simulink model "Tie_Line_bias"  (R2020a)
settings: Solver=VariableStepAuto  StartTime=0.0  StopTime=30  MaxStep=1e-4  RelTol=1e-3
libraries: powerlib x1
settings Model: Creator=Zebin  LastModifiedBy=Zebin

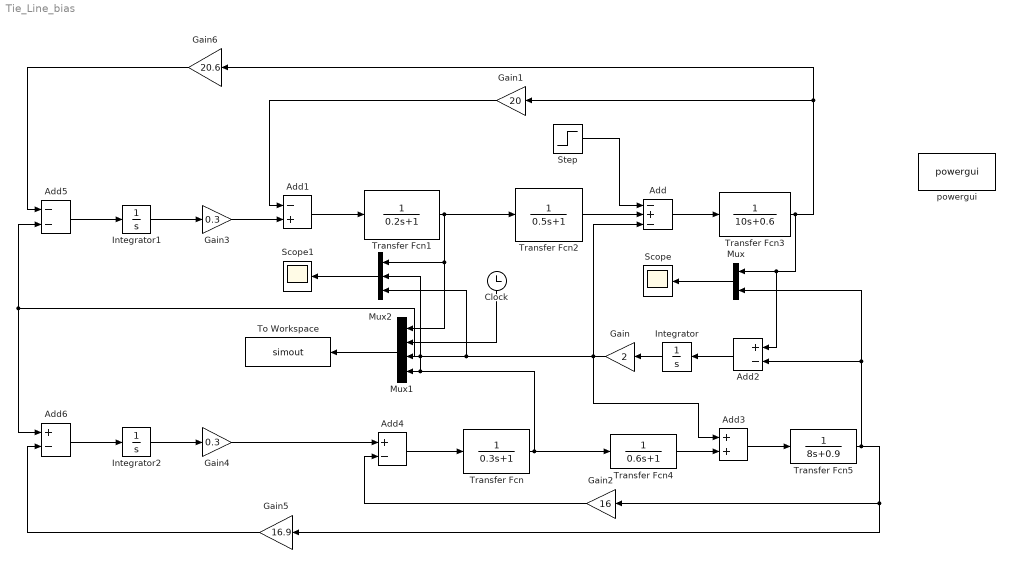
== system Tie_Line_bias ==
  Add : Sum  Inputs=-+-
  Add1 : Sum  Inputs=-+
  Add2 : Sum  Inputs=+-
  Add3 : Sum
  Add4 : Sum  Inputs=+-
  Add5 : Sum  Inputs=--
  Add6 : Sum  Inputs=+-
  "Clock " : Clock
  Gain : Gain  Gain=2
  Gain1 : Gain  Gain=20
  Gain2 : Gain  Gain=16
  Gain3 : Gain  Gain=0.3
  Gain4 : Gain  Gain=0.3
  Gain5 : Gain  Gain=16.9
  Gain6 : Gain  Gain=20.6
  Integrator : Integrator
  Integrator1 : Integrator
  Integrator2 : Integrator
  Mux : Mux  Inputs=2
  Mux1 : Mux
  Mux2 : Mux  Inputs=3
  Scope : Scope
  Scope1 : Scope
  Step : Step  Time=0  After=0.185  SampleTime=0
  To Workspace : ToWorkspace  VariableName=simout  SaveFormat=Timeseries  SampleTime=-1
  Transfer Fcn : TransferFcn  Denominator=[0.3 1]
  Transfer Fcn1 : TransferFcn  Denominator=[0.2 1]
  Transfer Fcn2 : TransferFcn  Denominator=[0.5 1]
  Transfer Fcn3 : TransferFcn  Denominator=[10 0.6]
  Transfer Fcn4 : TransferFcn  Denominator=[0.6 1]
  Transfer Fcn5 : TransferFcn  Denominator=[8 0.9]
  powergui : powerlib/powergui  Priority=1  SimulationMode=Continuous  SampleTime=50e-6  frequency=60  Iterations=50  frequencyindice=60  Pbase=100e6  ErrMax=1e-4  UnitsV=kV  UnitsW=MW  buscounter=0  FunctionMessages=off  echomessages=off  EnableUseOfTLC=off  CurrentSourceSwitches=off  DisableSnubberDevices=off  DisableRonSwitches=off  DisableVfSwitches=off  DisplayEquations=off  AutomaticDiscreteSolvers=off  SolverType=Tustin/Backward Euler (TBE)  Interpol=off  ExternalGateDelay=off  methode=off  Ts=100  x0status=blocks  SPID=on  SwTol=0  HookPort=off  NonlinearTolerance=1e-4  nMaxIteration=100  ContinueOnMaxIteration=off  RestoreLinks=warning  ResistiveCurrentMeasurement=off  Frange=[0:2:500]  Ylog=off  Xlog=on  ShowGrid=off  save=off  variable=ZData  structure=0  ZoomFFT=off  StartTime=0.0  cycles=1  DisplayStyle=1  fundamental=60  FreqAxis=off  MaxFrequency=1000  frequencyindicesteady=1  RmsSteady=1  display=off
  wires:
  Transfer Fcn1/1 -> Transfer Fcn2/1, Mux2/1, Mux1/1
  Transfer Fcn2/1 -> Add/2
  Step/1 -> Add/1
  Gain1/1 -> Add1/1
  Add/1 -> Transfer Fcn3/1
  Mux/1 -> Scope/1
  Add2/1 -> Integrator/1
  Integrator/1 -> Gain/1
  Add1/1 -> Transfer Fcn1/1
  "Clock "/1 -> Mux1/2
  Transfer Fcn/1 -> Mux2/2, Mux1/4, Transfer Fcn4/1
  Gain/1 -> Add/3, Add3/1, Mux2/3, Add6/1, Add5/2, Mux1/3
  Transfer Fcn4/1 -> Add3/2
  Add4/1 -> Transfer Fcn/1
  Add3/1 -> Transfer Fcn5/1
  Transfer Fcn5/1 -> Mux/2, Add2/2, Gain2/1, Gain5/1
  Mux1/1 -> To Workspace/1
  Mux2/1 -> Scope1/1
  Gain6/1 -> Add5/1
  Gain5/1 -> Add6/2
  Add6/1 -> Integrator2/1
  Integrator2/1 -> Gain4/1
  Gain2/1 -> Add4/2
  Gain4/1 -> Add4/1
  Add5/1 -> Integrator1/1
  Integrator1/1 -> Gain3/1
  Gain3/1 -> Add1/2
  Transfer Fcn3/1 -> Add2/1, Mux/1, Gain6/1, Gain1/1
